simulink model "untitled"  (R2023a)
settings: Solver=VariableStepAuto  StartTime=0.0  StopTime=40  RelTol=1e-3
settings Model: Creator=1  LastModifiedBy=刘侃
settings DebuggingCC: UnconnectedInputMsg=warning  UnconnectedOutputMsg=warning  UnconnectedLineMsg=warning
settings ModelReferenceCC: EnableRefExpFcnMdlSchedulingChecks=on
settings RTWCC: DLArmComputeVersion=19.05

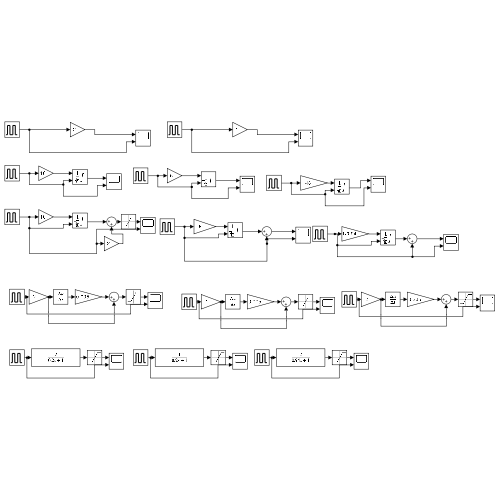
[thumbnail: Simulink's stored preview of the top-level diagram]
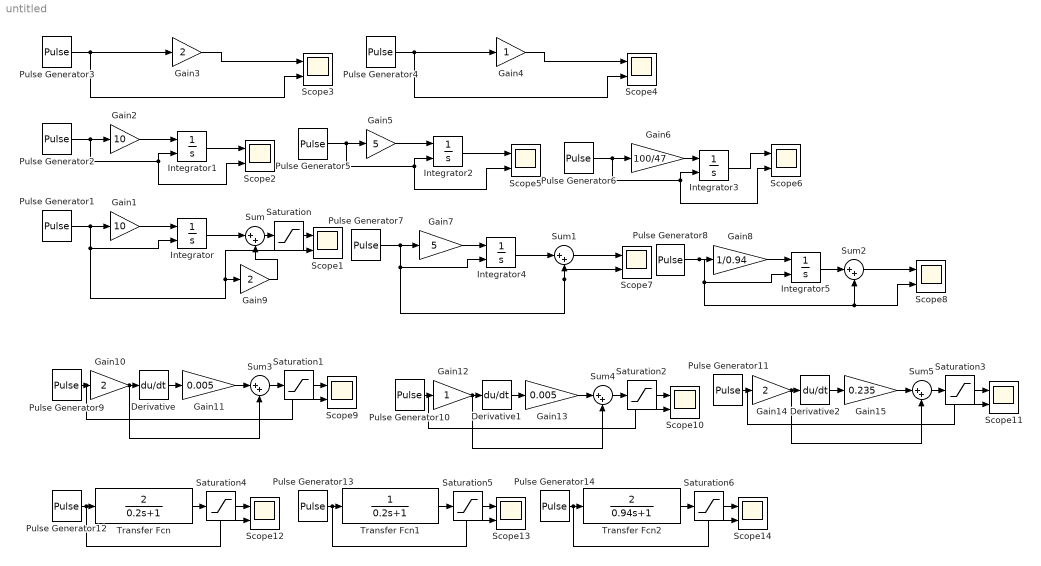
== system untitled ==
  Derivative : Derivative
  Derivative1 : Derivative
  Derivative2 : Derivative
  Gain1 : Gain  Gain=10
  Gain{3,9..10,14} (4 alike) : Gain  Gain=2
  Gain11 : Gain  Gain=0.005
  Gain12 : Gain
  Gain13 : Gain  Gain=0.005
  Gain15 : Gain  Gain=0.235
  Gain2 : Gain  Gain=10
  Gain4 : Gain
  Gain5 : Gain  Gain=5
  Gain6 : Gain  Gain=100/47
  Gain7 : Gain  Gain=5
  Gain8 : Gain  Gain=1/0.94
  Integrator : Integrator  ExternalReset=falling  LimitOutput=on  UpperSaturationLimit=10
  Integrator{1..5} (5 alike) : Integrator  ExternalReset=falling  LimitOutput=on  UpperSaturationLimit=9
  Pulse Generator1 : DiscretePulseGenerator  PulseType=Time based  Amplitude=5  PulseWidth=10  PhaseDelay=0.1
  Pulse Generator10 : DiscretePulseGenerator  PulseType=Time based  Amplitude=5  Period=1  PulseWidth=50  PhaseDelay=0.2
  Pulse Generator11 : DiscretePulseGenerator  PulseType=Time based  Amplitude=5  Period=1  PulseWidth=50  PhaseDelay=0.5
  Pulse Generator12 : DiscretePulseGenerator  PulseType=Time based  Amplitude=5  Period=9.1  PulseWidth=90  PhaseDelay=2
  Pulse Generator13 : DiscretePulseGenerator  PulseType=Time based  Amplitude=5  Period=9.1  PulseWidth=90  PhaseDelay=2
  Pulse Generator14 : DiscretePulseGenerator  PulseType=Time based  Amplitude=5  Period=9.1  PulseWidth=50  PhaseDelay=2
  Pulse Generator{2..6} (5 alike) : DiscretePulseGenerator  PulseType=Time based  Amplitude=5  Period=1  PulseWidth=50
  Pulse Generator7 : DiscretePulseGenerator  PulseType=Time based  Amplitude=5  PulseWidth=10  PhaseDelay=0.1
  Pulse Generator8 : DiscretePulseGenerator  PulseType=Time based  Amplitude=5  PulseWidth=10  PhaseDelay=0.1
  Pulse Generator9 : DiscretePulseGenerator  PulseType=Time based  Amplitude=5  Period=1  PulseWidth=50  PhaseDelay=0.2
  Saturation : Saturate  UpperLimit=9
  Saturation{1..2,4..6} (5 alike) : Saturate  UpperLimit=9  LowerLimit=-100
  Saturation3 : Saturate  UpperLimit=9
  Scope{1..14} (14 alike) : Scope  NumInputPorts=2
  Sum{,1..5} (6 alike) : Sum  Inputs=|++
  Transfer Fcn : TransferFcn  Numerator=[2]  Denominator=[0.2 1]
  Transfer Fcn1 : TransferFcn  Denominator=[0.2 1]
  Transfer Fcn2 : TransferFcn  Numerator=[2]  Denominator=[0.94 1]
  wires:
  Gain1/1 -> Integrator/1
  Integrator/1 -> Sum/1
  Pulse Generator1/1 -> Integrator/2, Gain9/1, Scope1/2, Gain1/1
  Pulse Generator2/1 -> Scope2/2, Integrator1/2, Gain2/1
  Integrator1/1 -> Scope2/1
  Gain2/1 -> Integrator1/1
  Pulse Generator3/1 -> Scope3/2, Gain3/1
  Gain3/1 -> Scope3/1
  Pulse Generator4/1 -> Scope4/2, Gain4/1
  Gain4/1 -> Scope4/1
  Integrator2/1 -> Scope5/1
  Pulse Generator5/1 -> Scope5/2, Integrator2/2, Gain5/1
  Gain5/1 -> Integrator2/1
  Integrator3/1 -> Scope6/1
  Pulse Generator6/1 -> Scope6/2, Integrator3/2, Gain6/1
  Gain6/1 -> Integrator3/1
  Integrator4/1 -> Sum1/1
  Pulse Generator7/1 -> Integrator4/2, Sum1/2, Scope7/2, Gain7/1
  Gain7/1 -> Integrator4/1
  Integrator5/1 -> Sum2/1
  Pulse Generator8/1 -> Integrator5/2, Scope8/2, Sum2/2, Gain8/1
  Gain8/1 -> Integrator5/1
  Gain9/1 -> Sum/2
  Sum/1 -> Saturation/1
  Saturation/1 -> Scope1/1
  Sum1/1 -> Scope7/1
  Sum2/1 -> Scope8/1
  Pulse Generator9/1 -> Scope9/2, Gain10/1
  Gain10/1 -> Derivative/1, Sum3/2
  Derivative/1 -> Gain11/1
  Gain11/1 -> Sum3/1
  Sum3/1 -> Saturation1/1
  Saturation1/1 -> Scope9/1
  Gain13/1 -> Sum4/1
  Saturation2/1 -> Scope10/1
  Gain12/1 -> Derivative1/1, Sum4/2
  Sum4/1 -> Saturation2/1
  Pulse Generator10/1 -> Scope10/2, Gain12/1
  Derivative1/1 -> Gain13/1
  Gain15/1 -> Sum5/1
  Saturation3/1 -> Scope11/1
  Gain14/1 -> Derivative2/1, Sum5/2
  Sum5/1 -> Saturation3/1
  Pulse Generator11/1 -> Scope11/2, Gain14/1
  Derivative2/1 -> Gain15/1
  Saturation4/1 -> Scope12/1
  Transfer Fcn/1 -> Saturation4/1
  Pulse Generator12/1 -> Scope12/2, Transfer Fcn/1
  Transfer Fcn1/1 -> Saturation5/1
  Saturation5/1 -> Scope13/1
  Pulse Generator13/1 -> Scope13/2, Transfer Fcn1/1
  Transfer Fcn2/1 -> Saturation6/1
  Saturation6/1 -> Scope14/1
  Pulse Generator14/1 -> Scope14/2, Transfer Fcn2/1
